simulink model "DynamicSimulation"  (R2017a)
settings: Solver=VariableStepAuto  StartTime=0.0  StopTime=10.0  RelTol=1e-3
values from neighbouring files (symbols this model uses):
  g = 9.8    [Parameters.m]
  L1 = 1    [Parameters.m]
  L2 = 0.8    [Parameters.m]
  m1 = 1    [Parameters.m]
  m2 = 0.8    [Parameters.m]
libraries: dspinverses x1
settings Model: Creator=adityaaaap  LastModifiedBy=adityaaaap

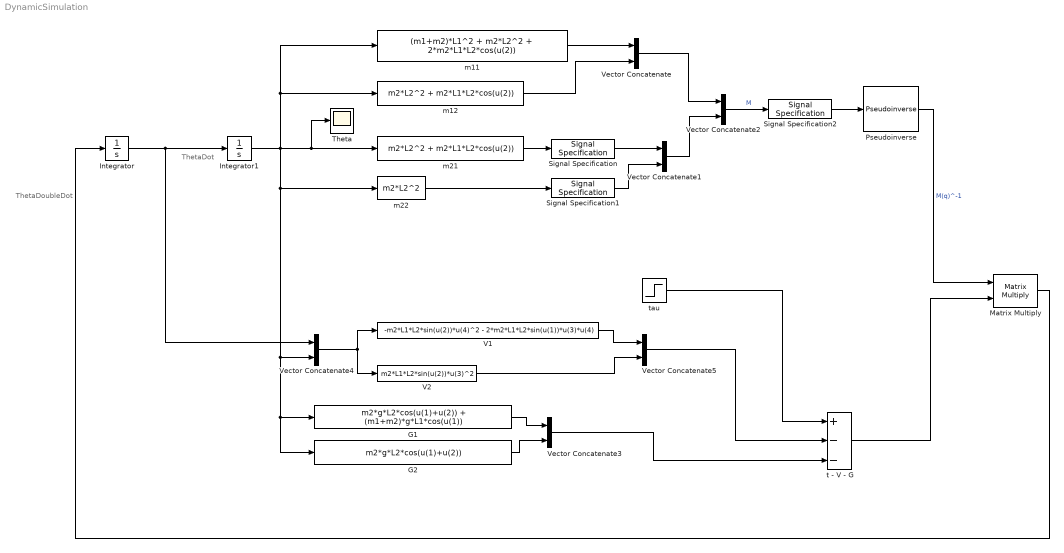
== system DynamicSimulation ==
  note: ThetaDoubleDot
  note: ThetaDot
  "G1 " : Fcn  Expr=m2*g*L2*cos(u(1)+u(2)) + (m1+m2)*g*L1*cos(u(1))
  G2 : Fcn  Expr=m2*g*L2*cos(u(1)+u(2))
  Integrator : Integrator
  Integrator1 : Integrator
  Matrix Multiply : Product  Multiplication=Matrix(*)
  Pseudoinverse : dspinverses/Pseudoinverse  wanterr=off  SimulateUsing=Interpreted execution
      settings: SourceProductName=DSP System Toolbox  SourceProductBaseCode=DS
  Signal Specification : SignalSpecification  Dimensions=[1,1]
  Signal Specification1 : SignalSpecification  Dimensions=[1,1]
  Signal Specification2 : SignalSpecification  Dimensions=[2,2]
  "Theta " : Scope
  "V1 " : Fcn  Expr=-m2*L1*L2*sin(u(2))*u(4)^2 - 2*m2*L1*L2*sin(u(1))*u(3)*u(4)
  V2 : Fcn  Expr=m2*L1*L2*sin(u(2))*u(3)^2
  Vector Concatenate : Concatenate  Mode=Multidimensional array  ConcatenateDimension=2
  Vector Concatenate1 : Concatenate  Mode=Multidimensional array  ConcatenateDimension=2
  Vector Concatenate2 : Concatenate  Mode=Multidimensional array
  Vector Concatenate3 : Concatenate  Mode=Multidimensional array
  Vector Concatenate4 : Concatenate
  Vector Concatenate5 : Concatenate
  "m11 " : Fcn  Expr=(m1+m2)*L1^2 + m2*L2^2 + 2*m2*L1*L2*cos(u(2))
  "m12 " : Fcn  Expr=m2*L2^2 + m2*L1*L2*cos(u(2))
  "m21 " : Fcn  Expr=m2*L2^2 + m2*L1*L2*cos(u(2))
  "m22 " : Fcn  Expr=m2*L2^2
  t - V - G : Sum  Inputs=+--
  "tau " : Step  SampleTime=0
  wires:
  "m21 "/1 -> Signal Specification/1
  Integrator1/1 -> "Theta "/1, "m21 "/1, "m12 "/1, "m11 "/1, G2/1, "G1 "/1, Vector Concatenate4/2, "m22 "/1
  Vector Concatenate4/1 -> V2/1, "V1 "/1
  Integrator/1 -> Integrator1/1, Vector Concatenate4/1
  "V1 "/1 -> Vector Concatenate5/1
  G2/1 -> Vector Concatenate3/2
  Matrix Multiply/1 -> Integrator/1
  "G1 "/1 -> Vector Concatenate3/1
  Signal Specification1/1 -> Vector Concatenate1/2
  "m12 "/1 -> Vector Concatenate/2
  Signal Specification2/1 -> Pseudoinverse/1
  "m22 "/1 -> Signal Specification1/1
  Signal Specification/1 -> Vector Concatenate1/1
  Vector Concatenate2/1 -> Signal Specification2/1  "M"
  Vector Concatenate1/1 -> Vector Concatenate2/2
  Pseudoinverse/1 -> Matrix Multiply/1  "M(q)^-1"
  "m11 "/1 -> Vector Concatenate/1
  t - V - G/1 -> Matrix Multiply/2
  Vector Concatenate/1 -> Vector Concatenate2/1
  "tau "/1 -> t - V - G/1
  Vector Concatenate3/1 -> t - V - G/3
  Vector Concatenate5/1 -> t - V - G/2
  V2/1 -> Vector Concatenate5/2
